simulink model "MainSim"  (R2025a)
settings: Solver=VariableStepAuto  StartTime=0.0  StopTime=110  MaxStep=0.01  RelTol=1e-3
undefined symbols (not defined in the file): bref, cref, g, inertia, m, m_carriage
libraries: fl_lib x79, nesl_utility x32, simulink_extras x9, sdl_lib x4, aerolibobsolete x2, ee_lib x2, slpidlib x2, aerolibadyn x1, matrix_library x1, aerolibatmos2 x1, aerolibwind2 x1, aerolibanim x1
(part 1 of 5)
settings Model: Creator=djangovanderplas  LastModifiedBy=djangovanderplas

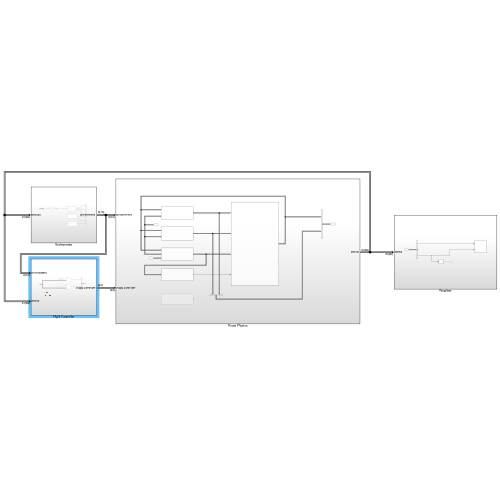
[thumbnail: Simulink's stored preview of the top-level diagram]
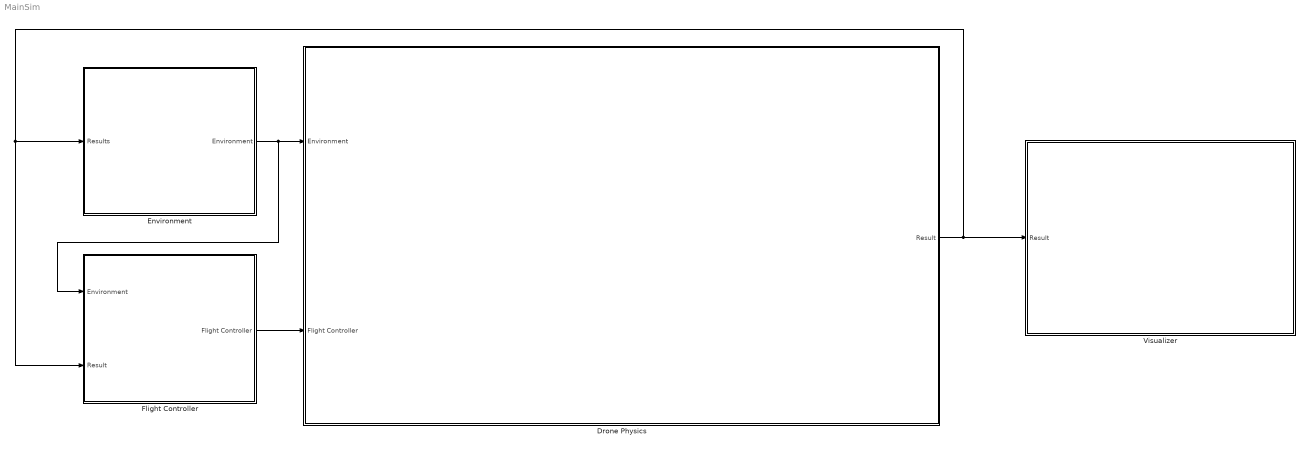
== system MainSim ==
  Drone Physics : Subsystem
  Environment : Subsystem
  Flight Controller : Subsystem
  Visualizer : Subsystem
  wires:
  Environment/1(Environment) -> Flight Controller/1(Environment), Drone Physics/1(Environment)
  Drone Physics/1(Result) -> Environment/1(Results), Flight Controller/2(Result), Visualizer/1(Result)
  Flight Controller/1(Flight Controller) -> Drone Physics/2(Flight Controller)

== system MainSim/Drone Physics ==
  Environment : Inport
  Flight Controller : Inport  Port=2
  Aerodynamics : Subsystem
  Bus Creator : BusCreator  Inputs=2
  Bus Creator1 : BusCreator  Inputs=2
  EoM : Subsystem  mask{X_BE0_E=[0 0 -500], V_BE0_B=[18 0 0], Eul_BL0=[0 deg2rad(10-1) deg2rad(0)], omega_dot_BL0_B=[7*2*pi 0*2*pi 0*2*pi], m=m, inertia=inertia, ground_level=0}
      mask prompts: X_BE0_E "Initial Position in Inertial(x_e, y_e, z_e) (m)"; V_BE0_B "Initial Velocity in Body (u, v, w) (m/s)"; Eul_BL0 "Initial Euler Angles (ψ, θ, φ) (rad)"; omega_dot_BL0_B "Initial Rotation Rates (p, q, r) (rad/s)"; m "Mass (kg)"; inertia "Inertia Tensor (kg⋅m2)"; ground_level "Ground Level (m)"
      mask DialogControl DescTextVar Prompt: Equations of Motion for the rotary drone
  Fake Force : Subsystem  Commented=on  mask{F_B=[0 0 0], M_B=[0 0 0], S_B=[0 0 0]}
      mask prompts: F_B "Body Force Vector (Fx, Fy, Fz) (N)"; M_B "Body Moment Vector (Mx, My, Mz) (Nm)"; S_B "Force moment arm (x, y, z) (m)"
  Gravity : Subsystem
  Propulsion : Subsystem
  Spring Model : Subsystem  mask{m_carriage=m_carriage, k=12.4, c=1, x_carriage_0=0.3*cref, x_n=0.5*cref, x_max=0.13103*cref, x_min=-0.21397*cref, x_cg_body=0.41757*cref}
      mask prompts: m_carriage "Carriage Mass (g)"; k "Spring Coefficient"; c "Damping Coefficient"; x_carriage_0 "Initial Location from LE (m)"; x_n "Natural Position from LE (m)"; x_max "Forward Limit"; x_min "Backward Limit"; x_cg_body "Body CG"
      mask DialogControl Container3 Prompt: Spring Parameters
      mask DialogControl Container4 Prompt: Body Parameters
  Result : Outport
  wires:
  Environment/1 -> Propulsion/2(Environment), Gravity/2(Environment), Aerodynamics/2(Environment)
  EoM/1(EoM) -> Propulsion/1(EoM), Gravity/1(EoM), Aerodynamics/1(EoM), Bus Creator/1  "EoM"
  Bus Creator/1 -> Result/1
  Bus Creator1/1 -> Bus Creator/2  "Forces"
  Gravity/1(Gravity) -> EoM/2(Gravity), Bus Creator1/1  "Gravity"
  Aerodynamics/1(Aerodynamics) -> EoM/1(Aerodynamics), Bus Creator1/2
  Propulsion/1(Propulsion) -> Spring Model/1(Propulsion), EoM/3(Propulsion)
  Flight Controller/1 -> Propulsion/3(Flight Controller)
  Spring Model/1(CG) -> EoM/4(CG)

== system MainSim/Environment ==
  Results : Inport
  Bus Creator : BusCreator  Inputs=6
  Bus Selector : BusSelector  OutputSignals=EoM.X_BE_E
  Gain : Gain  Gain=-1
  "Gravity " : Subsystem
  Lapse Rate Model : aerolibatmos2/ISA Atmosphere Model  useExtended=off  action=None  custom=on  viscosityOut=off  g=9.80665  gamma=1.4  R=287.0531  L=0.0065  h_trop=11000  h_strat=20000  rho0=1.225  P0=101325  T0=288.15  h0=0  S=110.4  Tref=273.15  muref=1.716e-05
      settings: LibrarySourceBlock=aerolibatmos2/Lapse Rate Model
  Selector : Selector  InputPortWidth=3  IndexOptions=Index vector (dialog)  Indices=[3]  OutputSizes=1
  Variant Subsystem : Subsystem  Variant=on  VariantControlMode=label  LabelModeActiveChoice=true
  Environment : Outport
  wires:
  Bus Creator/1 -> Environment/1
  Lapse Rate Model/4 -> Bus Creator/4  "rho"
  Lapse Rate Model/3 -> Bus Creator/3  "P"
  Lapse Rate Model/1 -> Bus Creator/1  "T_amb"
  "Gravity "/1(g_L) -> Bus Creator/5  "g_L"
  Lapse Rate Model/2 -> Bus Creator/2  "a"
  Variant Subsystem/1(V_wind) -> Bus Creator/6  "V_wind"
  Results/1 -> Bus Selector/1
  Selector/1 -> Gain/1
  Bus Selector/1 -> Selector/1  "<X_BE_E>"
  Gain/1 -> Lapse Rate Model/1

== system MainSim/Flight Controller ==
  Environment : Inport
  Result : Inport  Port=2
  Bus Creator : BusCreator  Inputs=2
  Roll Rate [Hz] : SliderBlock  ScaleMin=-20  ScaleMax=20
  Roll Regulator : Subsystem
  Slider : SliderBlock  ScaleMin=-10  ScaleMax=30
  Target Roll Rate [Hz] : Constant  Value=6.749226006191947
  Terminator : Terminator
  Theta Controller : Subsystem
  theta_target [deg] : Constant  Value=8.026315789473685
  Flight Controller : Outport
  wires:
  Result/1 -> Theta Controller/2(Result), Roll Regulator/2(Result)
  Environment/1 -> Terminator/1
  Bus Creator/1 -> Flight Controller/1
  Target Roll Rate [Hz]/1 -> Roll Regulator/1(roll_rate_target)  "roll_rate_target"
  Roll Regulator/1(differential) -> Bus Creator/2
  theta_target [deg]/1 -> Theta Controller/1(theta_target)  "theta_target"
  Theta Controller/1(throttle) -> Bus Creator/1  "throttle"

== system MainSim/Visualizer ==
  Result : Inport
  6DoF Animation : aerolibanim/6DoF Animation  u1=[0 4000 -2000 2000 -5000 -3000]  u2=1*1/25  u3=40  u4=[0 0 20]  u5=Fly alongside  u6=[50 50 -20]  u7=90  u8=on
  Bus Selector : BusSelector  OutputSignals=EoM.X_BE_E,EoM.V_BE_E,EoM.Eul_BL
  Radians to Degrees : simulink_extras/Transformations/Radians to Degrees
  wires:
  Result/1 -> Bus Selector/1
  Bus Selector/1 -> 6DoF Animation/1  "<X_BE_E>"
  Bus Selector/3 -> Radians to Degrees/1, 6DoF Animation/2  "<Eul_BL>"
  Radians to Degrees/1 -> ?  "Eul_Ang"

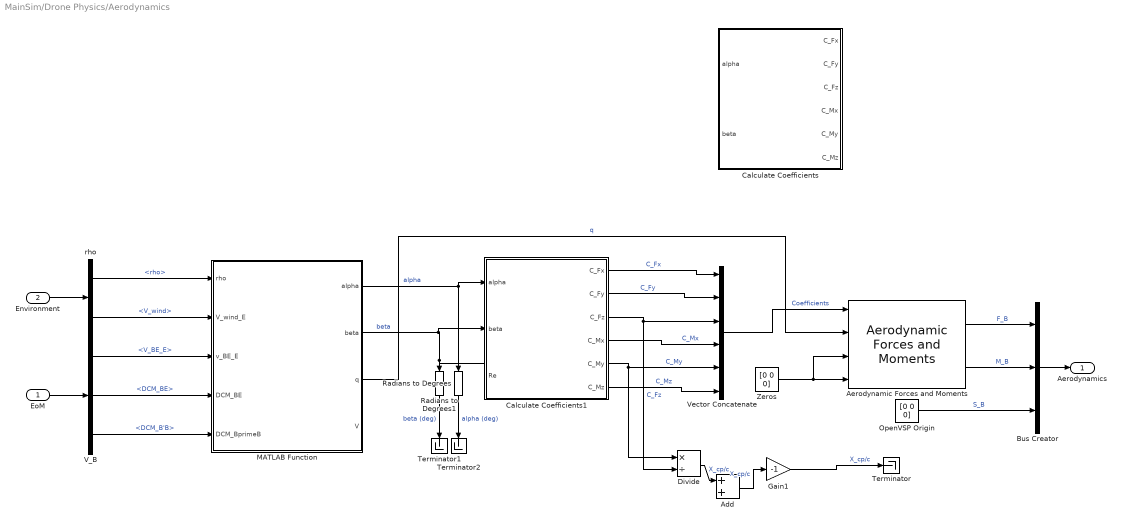
== system MainSim/Drone Physics/Aerodynamics ==
  EoM : Inport
  Environment : Inport  Port=2
  Add : Sum
  "Aerodynamic Forces and Moments " : aerolibadyn/Aerodynamic Forces and Moments   inputAxes=Body  outputForceAxes=Body  outputMomentAxes=Body  S=Sref  b=bref  cbar=cref
  Bus Creator : BusCreator  Inputs=3
  Calculate Coefficients : Subsystem
  Calculate Coefficients1 : Subsystem
  Divide : Product  Inputs=*/
  Gain1 : Gain  Gain=-1
  MATLAB Function : MATLAB Function  TreatAsAtomicUnit=on
  OpenVSP Origin : Constant  Value=[0 0 0]
  Radians to Degrees : simulink_extras/Transformations/Radians to Degrees
  Radians to Degrees1 : simulink_extras/Transformations/Radians to Degrees
  Terminator : Terminator
  Terminator1 : Terminator
  Terminator2 : Terminator
  V_B : BusSelector  OutputSignals=V_BE_E,DCM_BE,DCM_B'B
  Vector Concatenate : Concatenate  NumInputs=6
  Zeros : Constant  Value=[0 0 0]
  rho : BusSelector  OutputSignals=rho,V_wind
  Aerodynamics : Outport
  wires:
  EoM/1 -> V_B/1
  Environment/1 -> rho/1
  rho/1 -> MATLAB Function/1(rho)  "<rho>"
  rho/2 -> MATLAB Function/2(V_wind_E)  "<V_wind>"
  V_B/1 -> MATLAB Function/3(v_BE_E)  "<V_BE_E>"
  V_B/3 -> MATLAB Function/5(DCM_BprimeB)  "<DCM_B'B>"
  V_B/2 -> MATLAB Function/4(DCM_BE)  "<DCM_BE>"
  MATLAB Function/2(beta) -> Calculate Coefficients1/2(beta), Radians to Degrees1/1  "beta"
  MATLAB Function/1(alpha) -> Radians to Degrees/1, Calculate Coefficients1/1(alpha)  "alpha"
  Calculate Coefficients1/1(C_Fx) -> Vector Concatenate/1  "C_Fx"
  Calculate Coefficients1/2(C_Fy) -> Vector Concatenate/2  "C_Fy"
  Calculate Coefficients1/3(C_Fz) -> Vector Concatenate/3, Divide/2  "C_Fz"
  Calculate Coefficients1/4(C_Mx) -> Vector Concatenate/4  "C_Mx"
  Calculate Coefficients1/5(C_My) -> Vector Concatenate/5, Divide/1  "C_My"
  Calculate Coefficients1/6(C_Mz) -> Vector Concatenate/6  "C_Mz"
  MATLAB Function/3(q) -> "Aerodynamic Forces and Moments "/2  "q"
  Vector Concatenate/1 -> "Aerodynamic Forces and Moments "/1  "Coefficients"
  Add/1 -> Gain1/1  "X_cp/c"
  Radians to Degrees1/1 -> Terminator1/1  "beta (deg)"
  Radians to Degrees/1 -> Terminator2/1  "alpha (deg)"
  Zeros/1 -> "Aerodynamic Forces and Moments "/3, "Aerodynamic Forces and Moments "/4
  OpenVSP Origin/1 -> Bus Creator/3  "S_B"
  Bus Creator/1 -> Aerodynamics/1
  "Aerodynamic Forces and Moments "/2 -> Bus Creator/2  "M_B"
  "Aerodynamic Forces and Moments "/1 -> Bus Creator/1  "F_B"
  Gain1/1 -> Terminator/1  "X_cp/c"
  Divide/1 -> Add/1  "X_cp/c"

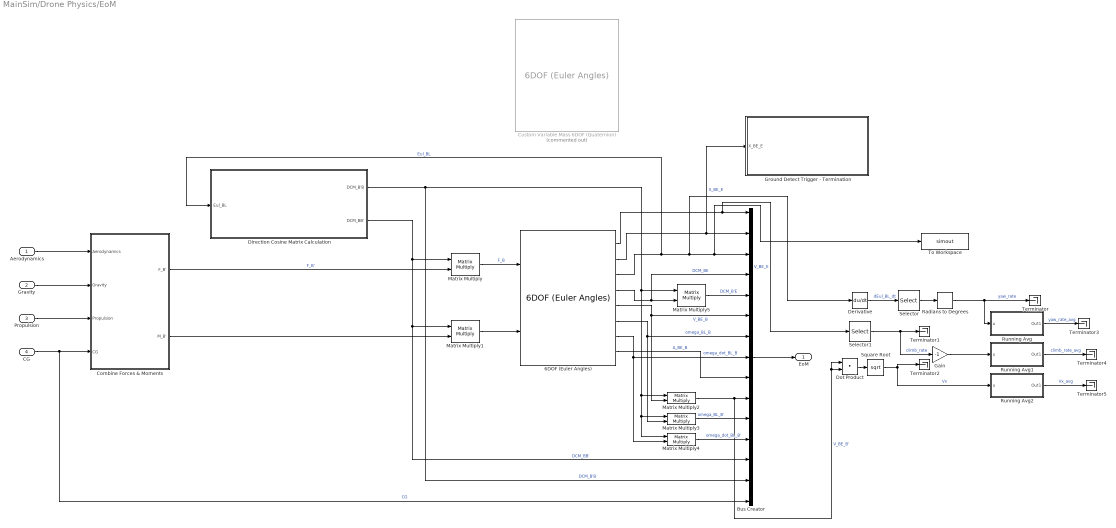
== system MainSim/Drone Physics/EoM ==
  Aerodynamics : Inport
  Gravity : Inport  Port=2
  Propulsion : Inport  Port=3
  CG : Inport  Port=4
  6DOF (Euler Angles) : aerolibobsolete/6DOF (Euler Angles)  units=Metric (MKS)  mtype=Fixed  rep=Quaternion  xme_0=X_BE0_E  Vm_0=V_BE0_B  eul_0=Eul_BL0  pm_0=omega_dot_BL0_B  mass_0=m  mass_e=0.5  mass_f=2.0  inertia=inertia  inertia_e=eye(3)  inertia_f=2*eye(3)  k_quat=1.0  vre_flag=on  abi_flag=off  aMode=0  xme_statename=''  Vm_statename=''  eul_statename=''  quat_statename=''  pm_statename=''  mass_statename=''
  Bus Creator : BusCreator  Inputs=15
  Combine Forces & Moments : Subsystem
  Custom Variable Mass 6DOF (Quaternion) : aerolibobsolete/6DOF (Euler Angles)  Commented=on  units=Metric (MKS)  mtype=Custom Variable  rep=Quaternion  xme_0=[0 0 0]  Vm_0=[0 0 0]  eul_0=[0 0 0]  pm_0=[0 0 0]  mass_0=1.0  mass_e=0.5  mass_f=2.0  inertia=eye(3)  inertia_e=eye(3)  inertia_f=2*eye(3)  k_quat=1.0  vre_flag=off  abi_flag=off  aMode=0  xme_statename=''  Vm_statename=''  eul_statename=''  quat_statename=''  pm_statename=''  mass_statename=''
  Derivative : Derivative
  Direction Cosine Matrix Calculation : Subsystem
  Dot Product : DotProduct  OutDataTypeStr=Inherit: Inherit via internal rule
  Gain : Gain  Gain=-1
  Ground Detect Trigger - Termination : Subsystem
  Matrix Multiply{,1..5} (6 alike) : Product  Multiplication=Matrix(*)
  Radians to Degrees : simulink_extras/Transformations/Radians to Degrees
  Running Avg : Subsystem
  Running Avg1 : Subsystem
  Running Avg2 : Subsystem
  Selector : Selector  InputPortWidth=3  IndexOptions=Index vector (dialog)  Indices=[3]  OutputSizes=1
  Selector1 : Selector  InputPortWidth=3  IndexOptions=Index vector (dialog)  Indices=[3]  OutputSizes=1
  Square Root : Sqrt
  Terminator{,1..5} (6 alike) : Terminator
  To Workspace : ToWorkspace  VariableName=simout  SaveFormat=Timeseries  SampleTime=-1
  EoM : Outport
  wires:
  6DOF (Euler Angles)/8 -> Bus Creator/9  "A_BE_B"
  Bus Creator/1 -> EoM/1
  6DOF (Euler Angles)/1 -> Selector1/1, Bus Creator/1  "V_BE_E"
  6DOF (Euler Angles)/4 -> Bus Creator/4, Matrix Multiply5/2  "DCM_BE"
  6DOF (Euler Angles)/3 -> Direction Cosine Matrix Calculation/1(Eul_BL), Derivative/1, To Workspace/1, Bus Creator/3  "Eul_BL"
  6DOF (Euler Angles)/7 -> Matrix Multiply4/2, Bus Creator/8  "omega_dot_BL_B"
  6DOF (Euler Angles)/2 -> Ground Detect Trigger - Termination/1(X_BE_E), Bus Creator/2  "X_BE_E"
  6DOF (Euler Angles)/5 -> Bus Creator/6, Matrix Multiply2/2  "V_BE_B"
  6DOF (Euler Angles)/6 -> Matrix Multiply3/2, Bus Creator/7  "omega_BL_B"
  Aerodynamics/1 -> Combine Forces & Moments/1(Aerodynamics)
  Gravity/1 -> Combine Forces & Moments/2(Gravity)
  Combine Forces & Moments/1(F_B') -> Matrix Multiply/2  "F_B'"
  Matrix Multiply2/1 -> Dot Product/2, Dot Product/1, Bus Creator/10  "V_BE_B'"
  Matrix Multiply3/1 -> Bus Creator/11  "omega_BL_B'"
  Matrix Multiply4/1 -> Bus Creator/12  "omega_dot_BL_B'"
  Direction Cosine Matrix Calculation/1(DCM_B'B) -> Bus Creator/14, Matrix Multiply5/1, Matrix Multiply4/1, Matrix Multiply3/1, Matrix Multiply2/1  "DCM_B'B"
  Direction Cosine Matrix Calculation/2(DCM_BB') -> Matrix Multiply/1, Bus Creator/13, Matrix Multiply1/1  "DCM_BB'"
  Matrix Multiply/1 -> 6DOF (Euler Angles)/1  "F_B"
  Matrix Multiply1/1 -> 6DOF (Euler Angles)/2
  Combine Forces & Moments/2(M_B') -> Matrix Multiply1/2
  Matrix Multiply5/1 -> Bus Creator/5  "DCM_B'E"
  CG/1 -> Bus Creator/15, Combine Forces & Moments/4(CG)  "CG"
  Propulsion/1 -> Combine Forces & Moments/3(Propulsion)
  Derivative/1 -> Selector/1  "dEul_BL_dt"
  Selector1/1 -> Gain/1, Terminator1/1  "climb_rate"
  Square Root/1 -> Terminator2/1, Running Avg2/1(u)  "Vx"
  Selector/1 -> Radians to Degrees/1
  Radians to Degrees/1 -> Running Avg/1(u), Terminator/1  "yaw_rate"
  Running Avg/1(Out1) -> Terminator3/1  "yaw_rate_avg"
  Running Avg1/1(Out1) -> Terminator4/1  "climb_rate_avg"
  Running Avg2/1(Out1) -> Terminator5/1  "Vx_avg"
  Gain/1 -> Running Avg1/1(u)
  Dot Product/1 -> Square Root/1

== system MainSim/Drone Physics/Fake Force ==
  Bus Creator : BusCreator  Inputs=3
  Constant : Constant  Value=F_B
  Constant1 : Constant  Value=M_B
  Constant2 : Constant  Value=S_B
  Fake Force : Outport
  wires:
  Constant2/1 -> Bus Creator/3  "S_B"
  Constant1/1 -> Bus Creator/2  "M_B"
  Constant/1 -> Bus Creator/1  "F_B"
  Bus Creator/1 -> Fake Force/1  "Fake Force"

== system MainSim/Drone Physics/Gravity ==
  EoM : Inport
  Environment : Inport  Port=2
  Bus Creator : BusCreator  Inputs=3
  Bus Selector : BusSelector  OutputSignals=g_L
  DCM_BE : BusSelector  OutputSignals=DCM_B'E
  Ground : Ground
  Ground1 : Ground
  Matrix Multiply : Product  Multiplication=Matrix(*)
  m_B : Gain  Gain=m
  Gravity : Outport
  wires:
  Environment/1 -> Bus Selector/1
  Bus Selector/1 -> m_B/1  "<g_L>"
  Bus Creator/1 -> Gravity/1
  EoM/1 -> DCM_BE/1
  Ground1/1 -> Bus Creator/3  "S_B"
  Matrix Multiply/1 -> Bus Creator/1  "F_B"
  Ground/1 -> Bus Creator/2  "M_B"
  DCM_BE/1 -> Matrix Multiply/1  "<DCM_B'E>"
  m_B/1 -> Matrix Multiply/2  "F_g_L"

== system MainSim/Drone Physics/Propulsion ==
  EoM : Inport
  Environment : Inport  Port=2
  Flight Controller : Inport  Port=3
  Bus Creator1 : BusCreator  Inputs=2
  Bus Selector : BusSelector  OutputSignals=throttle,differential
  Contra-Rotating Propeller : Subsystem  Commented=on
  Contra-Rotating Propeller1 : Subsystem
  ESC and Motor : Subsystem  Commented=on
  Mixer : MATLAB Function  TreatAsAtomicUnit=on
  Motor & ESC : Subsystem
  Motor & ESC1 : Subsystem
  Scope : Scope  NumInputPorts=2
      settings: ActiveDisplayYMinimum=-1  ActiveDisplayYMaximum=1  DataLoggingVariableName=ScopeData10
  Propulsion : Outport
  wires:
  Contra-Rotating Propeller1/2(M_B) -> Bus Creator1/2  "M_B"
  Mixer/2(Motor2_Command) -> Motor & ESC/1(Motor Signal), Scope/2  "Motor 2 Command"
  Contra-Rotating Propeller1/1(F_B) -> Bus Creator1/1  "F_B"
  Mixer/1(Motor1_Command) -> Motor & ESC1/1(Motor Signal), Scope/1  "Motor 1 Command"
  Bus Creator1/1 -> Propulsion/1
  Bus Selector/1 -> Mixer/1(Throttle_Command)  "<throttle>"
  Environment/1 -> Contra-Rotating Propeller1/1(Environment)
  Flight Controller/1 -> Bus Selector/1
  Bus Selector/2 -> Mixer/2(Roll_Command)  "<differential>"
  EoM/1 -> Contra-Rotating Propeller1/2(EoM)
  connections:
  Contra-Rotating Propeller1/LConn1 -- Motor & ESC1/RConn1
  Motor & ESC/RConn1 -- Contra-Rotating Propeller1/LConn2

== system MainSim/Drone Physics/Spring Model ==
  Propulsion : Inport
  Calculate CG : Subsystem
  Constant : Constant  Value=-x_cg_body
  Gain : Gain  Gain=1/cref
  Gain1 : Gain  Gain=1/cref
  Gain2 : Gain  Gain=1/cref
  Ground : Ground
  Spring : Subsystem
  Terminator : Terminator
  Terminator1 : Terminator
  Terminator2 : Terminator
  Vector Concatenate : Concatenate  NumInputs=3
  CG : Outport
  wires:
  Propulsion/1 -> Spring/1(Propulsion)
  Spring/1(x_cg_carriage1) -> Gain/1, Calculate CG/1(x_cg_carriage)  "x_cg_carriage"
  Vector Concatenate/1 -> CG/1
  Ground/1 -> Vector Concatenate/2, Vector Concatenate/3
  Gain/1 -> Terminator/1  "x_cg_carriage/C"
  Calculate CG/1(x_cg) -> Vector Concatenate/1, Gain1/1  "x_cg"
  Gain1/1 -> Terminator1/1  "x_cg/C"
  Constant/1 -> Calculate CG/2(x_cg_body), Gain2/1  "x_cg_body"
  Gain2/1 -> Terminator2/1  "x_cg_body/C"

== system MainSim/Environment/Gravity  ==
  Constant : Constant  Value=[0 0 g]
  g_L : Outport
  wires:
  Constant/1 -> g_L/1

== system MainSim/Environment/Variant Subsystem ==
  note: 1) Add Subsystem or Model blocks as valid variant choices.
      | 2) You cannot connect blocks at this level. At simulation, connectivity is automatically
      | determined, based on the active variant and port name matching.
  V (m/s) : Inport
  Constant Wind : Subsystem  VariantControl=true  mask{v_wind_x=0, v_wind_y=0, v_wind_z=0}
      mask prompts: v_wind_x "V wind x"; v_wind_y "V wind y"; v_wind_z "V wind z"
      mask DialogControl DescTextVar Prompt: Test
  Discrete Gust : Subsystem  VariantControl=false
  V_wind : Outport

== system MainSim/Flight Controller/Roll Regulator ==
  roll_rate_target : Inport
  Result : Inport  Port=2
  Bus Selector : BusSelector  OutputSignals=EoM.omega_BL_B
  Gain : Gain  Gain=-1
  Gain1 : Gain  Gain=2*pi
  PID Controller : slpidlib/PID Controller  Controller=PID  Form=Parallel  TimeDomain=Continuous-time  UseExternalTs=off  SampleTime=-1  IntegratorMethod=Forward Euler  FilterMethod=Forward Euler  ControllerParametersSource=internal  P=100  I=2  UseKiTs=off  D=0  UseExternalDerivativeSource=off  N=100  UseFilter=on  TunerSelectOption=Transfer Function Based (PID Tuner App)  InitialConditionSource=internal  InitialConditionForIntegrator=0  InitialConditionForFilter=0  DifferentiatorICPrevScaledInput=0  ExternalReset=none  TrackingMode=off  Kt=1  LimitOutput=on  SatLimitsSource=internal  UpperSaturationLimit=1  LowerSaturationLimit=-1  LinearizeAsGain=on  AntiWindupMode=none  Kb=1  LimitIntegrator=off  UpperIntegratorSaturationLimit=inf  LowerIntegratorSaturationLimit=-inf  POutMin=[]  POutMax=[]  IOutMin=[]  IOutMax=[]  DOutMin=[]  DOutMax=[]  NOutMin=[]  NOutMax=[]  SumOutMin=[]  SumOutMax=[]  SaturationOutMin=[]  SaturationOutMax=[]  PParamMin=[]  PParamMax=[]  IParamMin=[]  IParamMax=[]  DParamMin=[]  DParamMax=[]  NParamMin=[]  NParamMax=[]  KbParamMin=[]  KbParamMax=[]  KtParamMin=[]  KtParamMax=[]  KbOutMin=[]  KbOutMax=[]  KtOutMin=[]  KtOutMax=[]  IntegratorOutMin=[]  IntegratorOutMax=[]  FilterOutMin=[]  FilterOutMax=[]  SumI1OutMin=[]  SumI1OutMax=[]  SumI2OutMin=[]  SumI2OutMax=[]  SumI3OutMin=[]  SumI3OutMax=[]  SumI4OutMin=[]  SumI4OutMax=[]  SumDOutMin=[]  SumDOutMax=[]  DifferentiatorOutMin=[]  DifferentiatorOutMax=[]  FilterDiffOutCoefMin=[]  FilterDiffOutCoefMax=[]  ReciprocalOutMin=[]  ReciprocalOutMax=[]  SumDenOutMin=[]  SumDenOutMax=[]  SumNumOutMin=[]  SumNumOutMax=[]  DivideOutMin=[]  DivideOutMax=[]  UdiffTsProdOutMin=[]  UdiffTsProdOutMax=[]  NTsProdOutMin=[]  NTsProdOutMax=[]  UintegralTsProdOutMin=[]  UintegralTsProdOutMax=[]  UngainTsProdOutMin=[]  UngainTsProdOutMax=[]  ClampingZeroOutDataTypeStr=Inherit: Inherit via back propagation  ClampingZeroOutMin=[]  ClampingZeroOutMax=[]  FilterDenConstantOutDataTypeStr=Inherit: Inherit via back propagation  FilterDenConstantOutMin=[]  FilterDenConstantOutMax=[]  PCopyOutDataTypeStr=Inherit: Inherit via back propagation  PCopyOutMin=[]  PCopyOutMax=[]  NCopyOutDataTypeStr=Inherit: Inherit via back propagation  NCopyOutMin=[]  NCopyOutMax=[]  IntegratorContinuousStateAttributes=''  IntegratorStateMustResolveToSignalObject=off  IntegratorRTWStateStorageClass=Auto  FilterContinuousStateAttributes=''  FilterStateMustResolveToSignalObject=off  FilterRTWStateStorageClass=Auto  ParallelPVariant=InternalParameters  IdealPVariant=Disabled  IVariant=InternalParameters  DVariant=InternalParameters  IntegratorVariant=Continuous  SatVariant=Enabled  AWVariant=Passthrough  PCopyVariant=Disabled  TRVariant=Disabled  FdbkBlocksVariant=Forward  IdealPFdbkVariant=Disabled  SatFdbkVariant=Disabled  DerivativeFilterVariant=ContFilter  NVariant=InternalParameters  NCopyVariant=Disabled  FilterICVariant=InternalICsFilter  IntegratorICVariant=InternalICs  ExternalResetVariant=Disabled  TRSumVariant=Passthrough  SumFdbkVariant=Disabled  SumVariant=Sum_PID  TsampFilterVariant=InternalTs  TsampNgainVariant=Passthrough  TsampIntegralVariant=Disabled_SignalSpec  ExternalSaturationOutDataTypeStr=Inherit: Same as second input  DerivativeSourceVariant=ErrorSignal  PreIntVariant=InternalPreInt
  Selector : Selector  InputPortWidth=3  IndexOptions=Index vector (dialog)  Indices=[1 ]  OutputSizes=1
  Sum : Sum  Inputs=|+-
  differential : Outport
  wires:
  roll_rate_target/1 -> Gain1/1
  Selector/1 -> Sum/2  "roll_rate_result"
  Result/1 -> Bus Selector/1
  Sum/1 -> PID Controller/1  "roll_rate_error"
  Bus Selector/1 -> Selector/1  "<omega_BL_B>"
  Gain/1 -> differential/1  "differential"
  PID Controller/1 -> Gain/1  "differential"
  Gain1/1 -> Sum/1

== system MainSim/Flight Controller/Theta Controller ==
  theta_target : Inport
  Result : Inport  Port=2
  Bus Selector1 : BusSelector  OutputSignals=EoM.Eul_BL
  Gain1 : Gain  Gain=-1
  PID Controller1 : slpidlib/PID Controller  Controller=PID  Form=Parallel  TimeDomain=Continuous-time  UseExternalTs=off  SampleTime=-1  IntegratorMethod=Forward Euler  FilterMethod=Forward Euler  ControllerParametersSource=internal  P=0.04  I=0.03  UseKiTs=off  D=0.01  UseExternalDerivativeSource=off  N=100  UseFilter=on  TunerSelectOption=Transfer Function Based (PID Tuner App)  InitialConditionSource=internal  InitialConditionForIntegrator=0  InitialConditionForFilter=0  DifferentiatorICPrevScaledInput=0  ExternalReset=none  TrackingMode=off  Kt=1  LimitOutput=on  SatLimitsSource=internal  UpperSaturationLimit=2  LowerSaturationLimit=0  LinearizeAsGain=off  AntiWindupMode=none  Kb=1  LimitIntegrator=off  UpperIntegratorSaturationLimit=inf  LowerIntegratorSaturationLimit=-inf  POutMin=[]  POutMax=[]  IOutMin=[]  IOutMax=[]  DOutMin=[]  DOutMax=[]  NOutMin=[]  NOutMax=[]  SumOutMin=[]  SumOutMax=[]  SaturationOutMin=[]  SaturationOutMax=[]  PParamMin=[]  PParamMax=[]  IParamMin=[]  IParamMax=[]  DParamMin=[]  DParamMax=[]  NParamMin=[]  NParamMax=[]  KbParamMin=[]  KbParamMax=[]  KtParamMin=[]  KtParamMax=[]  KbOutMin=[]  KbOutMax=[]  KtOutMin=[]  KtOutMax=[]  IntegratorOutMin=[]  IntegratorOutMax=[]  FilterOutMin=[]  FilterOutMax=[]  SumI1OutMin=[]  SumI1OutMax=[]  SumI2OutMin=[]  SumI2OutMax=[]  SumI3OutMin=[]  SumI3OutMax=[]  SumI4OutMin=[]  SumI4OutMax=[]  SumDOutMin=[]  SumDOutMax=[]  DifferentiatorOutMin=[]  DifferentiatorOutMax=[]  FilterDiffOutCoefMin=[]  FilterDiffOutCoefMax=[]  ReciprocalOutMin=[]  ReciprocalOutMax=[]  SumDenOutMin=[]  SumDenOutMax=[]  SumNumOutMin=[]  SumNumOutMax=[]  DivideOutMin=[]  DivideOutMax=[]  UdiffTsProdOutMin=[]  UdiffTsProdOutMax=[]  NTsProdOutMin=[]  NTsProdOutMax=[]  UintegralTsProdOutMin=[]  UintegralTsProdOutMax=[]  UngainTsProdOutMin=[]  UngainTsProdOutMax=[]  ClampingZeroOutDataTypeStr=Inherit: Inherit via back propagation  ClampingZeroOutMin=[]  ClampingZeroOutMax=[]  FilterDenConstantOutDataTypeStr=Inherit: Inherit via back propagation  FilterDenConstantOutMin=[]  FilterDenConstantOutMax=[]  PCopyOutDataTypeStr=Inherit: Inherit via back propagation  PCopyOutMin=[]  PCopyOutMax=[]  NCopyOutDataTypeStr=Inherit: Inherit via back propagation  NCopyOutMin=[]  NCopyOutMax=[]  IntegratorContinuousStateAttributes=''  IntegratorStateMustResolveToSignalObject=off  IntegratorRTWStateStorageClass=Auto  FilterContinuousStateAttributes=''  FilterStateMustResolveToSignalObject=off  FilterRTWStateStorageClass=Auto  ParallelPVariant=InternalParameters  IdealPVariant=Disabled  IVariant=InternalParameters  DVariant=InternalParameters  IntegratorVariant=Continuous  SatVariant=Enabled  AWVariant=Passthrough  PCopyVariant=Disabled  TRVariant=Disabled  FdbkBlocksVariant=Forward  IdealPFdbkVariant=Disabled  SatFdbkVariant=Disabled  DerivativeFilterVariant=ContFilter  NVariant=InternalParameters  NCopyVariant=Disabled  FilterICVariant=InternalICsFilter  IntegratorICVariant=InternalICs  ExternalResetVariant=Disabled  TRSumVariant=Passthrough  SumFdbkVariant=Disabled  SumVariant=Sum_PID  TsampFilterVariant=InternalTs  TsampNgainVariant=Passthrough  TsampIntegralVariant=Disabled_SignalSpec  ExternalSaturationOutDataTypeStr=Inherit: Same as second input  DerivativeSourceVariant=ErrorSignal  PreIntVariant=InternalPreInt
  Radians to Degrees : simulink_extras/Transformations/Radians to Degrees
  Selector1 : Selector  InputPortWidth=3  IndexOptions=Index vector (dialog)  Indices=[2]  OutputSizes=1
  Sum1 : Sum  Inputs=-+|
  throttle : Outport
  wires:
  theta_target/1 -> Sum1/2
  PID Controller1/1 -> throttle/1  "throttle"
  Gain1/1 -> PID Controller1/1
  Bus Selector1/1 -> Selector1/1  "<Eul_BL>"
  Selector1/1 -> Radians to Degrees/1  "theta_result"
  Radians to Degrees/1 -> Sum1/1  "theta_result"
  Result/1 -> Bus Selector1/1
  Sum1/1 -> Gain1/1  "x_cg_error"
